simulink model "MLI"  (R2013a)
settings: Solver=ode45  StartTime=0.0  StopTime=0.001  RelTol=1e-3
libraries: simulink x1
settings Model: Creator=DELL  LastModifiedBy=DELL

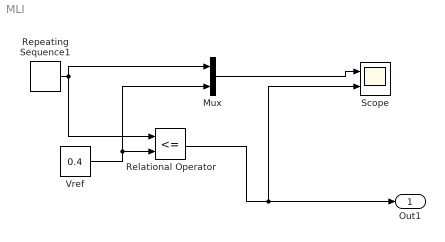
== system MLI ==
  Mux : Mux  Inputs=2
  Relational Operator : RelationalOperator  Operator=<=  OutDataTypeStr=boolean
  Repeating Sequence1 : simulink/Sources/Repeating Sequence  rep_seq_t=[0 (1/20000) (1/10000)]  rep_seq_y=[0 1 0]
  Scope : Scope  NumInputPorts=2
      settings: YMin=-5~-5  YMax=5~5
  Vref : Constant  Value=0.4
  Out1 : Outport
  wires:
  Vref/1 -> Relational Operator/2, Mux/2
  Relational Operator/1 -> Scope/2, Out1/1
  Mux/1 -> Scope/1
  Repeating Sequence1/1 -> Mux/1, Relational Operator/1
